simulink model "FMLibrary_v2_progress"  (R2016b)
settings: Solver=VariableStepAuto  StartTime=0.0  StopTime=10.0  RelTol=1e-3
undefined symbols (not defined in the file or in its folder): Lb, Lf, Lu, RobotStruct, sampleTime
libraries: simulink x24, FM_Library x10, VariousBlocksLibrary x10, FMLibrary_v2 x2, simulink_extras x2
(part 2 of 3)

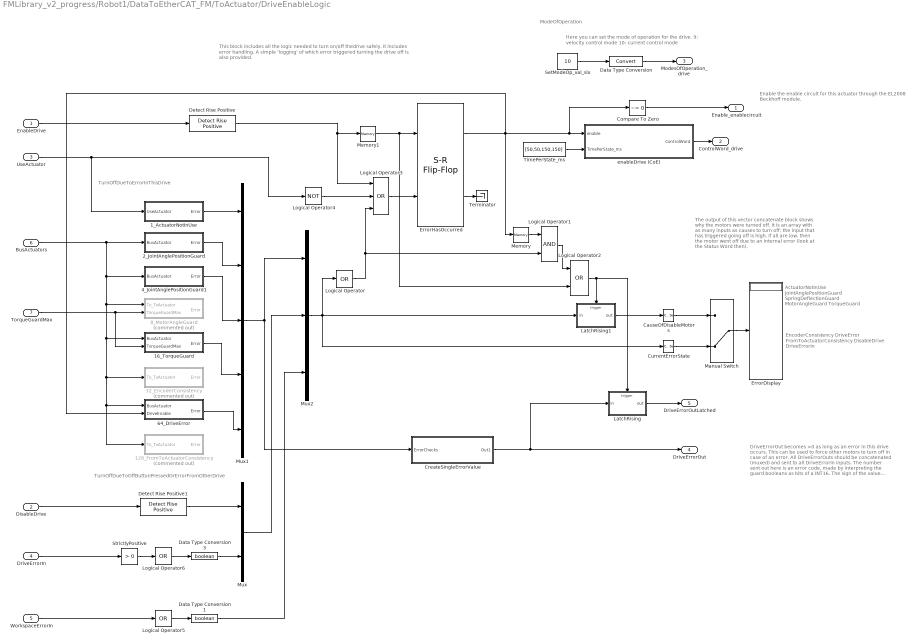
== system FMLibrary_v2_progress/Robot1/DataToEtherCAT_FM/ToActuator/DriveEnableLogic ==
  note: Here you can set the mode of operation for the drive.
      | 9: velocity control mode
      | 10: current control mode
  note: The output of this vector concatenate block shows why the motors were turned off. It is an array with as many inputs as causes to turn off; the input that has triggered going off is high. If all are low, then the motor went off due to an internal error (look at the Status Word then).
  note: This block includes all the logic needed to turn on/off thedrive safely. It includes error handling. A simple 'logging' of which error triggered turning the drive off is also provided.
  note: TurnOffDueToErrorInThisDrive
  note: TurnOffDueToOffButtonPressedOrErrorFromOtherDrive
  note: DriveErrorOut becomes >0 as long as an error in this drive occurs. This can be used to force other motors to turn off in case of an error.
      | All DriveErrorOuts should be concatenated (muxed)  and sent to all DriveErrorIn inputs. The number sent out here is an error code, made by interpreting the guard booleans as bits of a INT16.
      | The sign of the value indicates:
      | >=0: UseActuator=true
      | <0: UseActuator = False
  note: EncoderConsistency
      | DriveError
      | FromToActuatorConsistency
      | DisableDrive
      | DriveErrorIn
  note: ActuatorNotInUse
      | JointAnglePositionGuard
      | SpringDeflectionGuard
      | MotorAngleGuard
      | TorqueGuard
  note: ModeOfOperation
  note: Enable the enable circuit for this actuator through the EL2008
      | Beckhoff module.
  EnableDrive : Inport
  DisableDrive : Inport  Port=2
  UseActuator : Inport  Port=3
  DriveErrorIn : Inport  Port=4
  WorkspaceErrorIn : Inport  Port=5
  BusActuators : Inport  Port=6
  TorqueGuardMax : Inport  Port=7
  128_FromToActuatorConsistency : Subsystem  Commented=on
  16_TorqueGuard : Subsystem
  1_ActuatorNotInUse : Subsystem
  2_JointAnglePositionGuard : Subsystem
  32_EncoderConsistency : Subsystem  Commented=on
  4_JointAnglePositionGuard1 : Subsystem
  64_DriveError : Subsystem
  8_MotorAngleGuard : Subsystem  Commented=on
  CauseOfDisableMotors : Concatenate  NumInputs=1
  Compare To Zero : simulink/Logic and Bit Operations/Compare To Zero  relop=~=  OutDataTypeStr=boolean
  CreateSingleErrorValue : Subsystem
  CurrentErrorState : Concatenate  NumInputs=1
  Data Type Conversion : DataTypeConversion
  Data Type Conversion1 : DataTypeConversion  OutDataTypeStr=boolean
  Data Type Conversion3 : DataTypeConversion  OutDataTypeStr=boolean
  Detect Rise Positive : simulink/Logic and Bit Operations/Detect Rise Positive  vinit=0  InputProcessing=Inherited  OutDataTypeStr=boolean
  Detect Rise Positive1 : simulink/Logic and Bit Operations/Detect Rise Positive  vinit=0  InputProcessing=Inherited  OutDataTypeStr=boolean
  ErrorDisplay : Display
  ErrorHasOccurred : simulink_extras/Flip Flops/S-R Flip-Flop  initial_condition=0
  LatchRising : Subsystem  TreatAsAtomicUnit=on
  LatchRising1 : Subsystem  TreatAsAtomicUnit=on
  Logical Operator : Logic  Operator=OR  Inputs=1  AllPortsSameDT=off  OutDataTypeStr=boolean
  Logical Operator1 : Logic  AllPortsSameDT=off  OutDataTypeStr=boolean
  Logical Operator2 : Logic  Operator=OR  AllPortsSameDT=off  OutDataTypeStr=boolean
  Logical Operator3 : Logic  Operator=OR  Inputs=3  AllPortsSameDT=off  OutDataTypeStr=boolean
  Logical Operator4 : Logic  Operator=NOT  Inputs=1  AllPortsSameDT=off  OutDataTypeStr=boolean
  Logical Operator5 : Logic  Operator=OR  Inputs=1  AllPortsSameDT=off  OutDataTypeStr=boolean
  Logical Operator6 : Logic  Operator=OR  Inputs=1  AllPortsSameDT=off  OutDataTypeStr=boolean
  Manual Switch : ManualSwitch  CurrentSetting=0
  Memory : Memory
  Memory1 : Memory
  Mux : Mux  Inputs=2
  Mux1 : Mux  Inputs=5
  Mux2 : Mux  Inputs=3
  SetModeOp_val_slx : Constant  Value=10
  StrictlyPositive : simulink/Logic and Bit Operations/Compare To Zero  relop=>  OutDataTypeStr=boolean
  Terminator : Terminator
  TimePerState_ms : Constant  Value=[50,50,150,150]
  enableDrive (CoE) : MATLAB Function  TreatAsAtomicUnit=on
  Enable_enablecircuit : Outport
  ControlWord_drive : Outport  Port=2
  ModesOfOperation_drive : Outport  Port=3
  DriveErrorOut : Outport  Port=4
  DriveErrorOutLatched : Outport  Port=5
  wires:
  Data Type Conversion1/1 -> Mux2/3
  Mux1/1 -> Mux2/1, CreateSingleErrorValue/1(ErrorChecks)
  WorkspaceErrorIn/1 -> Logical Operator5/1
  Logical Operator5/1 -> Data Type Conversion1/1
  Data Type Conversion3/1 -> Mux/2
  Compare To Zero/1 -> Enable_enablecircuit/1
  16_TorqueGuard/1(Error) -> Mux1/4
  64_DriveError/1(Error) -> Mux1/5
  1_ActuatorNotInUse/1(Error) -> Mux1/1
  Logical Operator4/1 -> Logical Operator3/2
  BusActuators/1 -> 4_JointAnglePositionGuard1/1(BusActuator), 32_EncoderConsistency/1(To_ToActuator), 64_DriveError/1(BusActuator), 128_FromToActuatorConsistency/1(To_ToActuator), 16_TorqueGuard/1(BusActuator), 8_MotorAngleGuard/1(To_ToActuator), 2_JointAnglePositionGuard/1(BusActuator)
  Mux/1 -> Mux2/2
  Logical Operator6/1 -> Data Type Conversion3/1
  DriveErrorIn/1 -> StrictlyPositive/1
  UseActuator/1 -> Logical Operator4/1, 1_ActuatorNotInUse/1(UseActuator)
  TimePerState_ms/1 -> enableDrive (CoE)/2(TimePerState_ms)
  Detect Rise Positive/1 -> Memory1/1, Logical Operator3/1
  Logical Operator3/1 -> ErrorHasOccurred/2
  Manual Switch/1 -> ErrorDisplay/1
  Logical Operator1/1 -> Logical Operator2/1
  CurrentErrorState/1 -> Manual Switch/2
  Logical Operator2/1 -> LatchRising/Trigger, LatchRising1/Trigger
  Memory/1 -> Logical Operator1/1
  Memory1/1 -> ErrorHasOccurred/1, Logical Operator2/2
  CauseOfDisableMotors/1 -> Manual Switch/1
  Data Type Conversion/1 -> ModesOfOperation_drive/1
  ErrorHasOccurred/2 -> Terminator/1
  DisableDrive/1 -> Detect Rise Positive1/1
  Detect Rise Positive1/1 -> Mux/1
  Mux2/1 -> LatchRising1/1(in), CurrentErrorState/1, Logical Operator/1
  ErrorHasOccurred/1 -> enableDrive (CoE)/1(enable), Compare To Zero/1, 64_DriveError/2(DriveEnable), Memory/1
  enableDrive (CoE)/1(ControlWord) -> ControlWord_drive/1
  EnableDrive/1 -> Detect Rise Positive/1
  SetModeOp_val_slx/1 -> Data Type Conversion/1
  Logical Operator/1 -> Logical Operator1/2, Logical Operator3/3
  LatchRising1/1(out) -> CauseOfDisableMotors/1
  TorqueGuardMax/1 -> 8_MotorAngleGuard/2(TorqueGuardMax), 16_TorqueGuard/2(TorqueGuardMax)
  StrictlyPositive/1 -> Logical Operator6/1
  CreateSingleErrorValue/1(Out1) -> LatchRising/1(in), DriveErrorOut/1
  LatchRising/1(out) -> DriveErrorOutLatched/1
  4_JointAnglePositionGuard1/1(Error) -> Mux1/3
  2_JointAnglePositionGuard/1(Error) -> Mux1/2

== system FMLibrary_v2_progress/Robot1/DataToEtherCAT_FM/ToActuator1/AppendToBus ==
  Bus_in : Inport
  DriveError : Inport  Port=2
  DesiredTorque : Inport  Port=3
  DesiredTorqueLimited : Inport  Port=4
  Bus Creator : BusCreator  Inputs=12
  Bus Selector2 : BusSelector  OutputSignals=OperationEnabled,StatusWord,JointPosition_rad,JointVelocity_rads,MotorEncoder_counts,MotorPosition_IncEnc_rad,JointPosition_IncEnc_rad,JointAbsoluteEncoder_counts,JointTorque_Act_Nm
  Data Type Conversion : DataTypeConversion  OutDataTypeStr=double
  Bus_out : Outport
  wires:
  Bus Selector2/9 -> Bus Creator/9  "<JointTorque_Act_Nm>"
  Bus Creator/1 -> Bus_out/1
  Bus_in/1 -> Bus Selector2/1
  DriveError/1 -> Data Type Conversion/1
  Data Type Conversion/1 -> Bus Creator/12  "DriveError"
  DesiredTorque/1 -> Bus Creator/10  "DesiredTorque_Nm"
  DesiredTorqueLimited/1 -> Bus Creator/11  "DesiredTorqueLimited_Nm"
  Bus Selector2/1 -> Bus Creator/1  "<OperationEnabled>"
  Bus Selector2/2 -> Bus Creator/2  "<StatusWord>"
  Bus Selector2/3 -> Bus Creator/3  "<JointPosition_rad>"
  Bus Selector2/4 -> Bus Creator/4  "<JointVelocity_rads>"
  Bus Selector2/5 -> Bus Creator/5  "<MotorEncoder_counts>"
  Bus Selector2/7 -> Bus Creator/7  "<JointPosition_IncEnc_rad>"
  Bus Selector2/8 -> Bus Creator/8  "<JointAbsoluteEncoder_counts>"
  Bus Selector2/6 -> Bus Creator/6  "<MotorPosition_IncEnc_rad>"

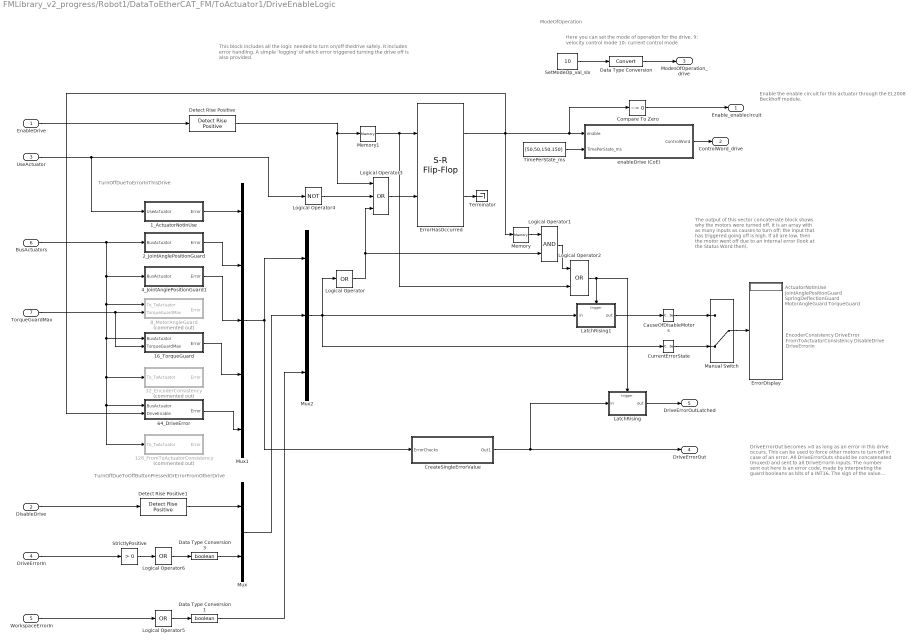
== system FMLibrary_v2_progress/Robot1/DataToEtherCAT_FM/ToActuator1/DriveEnableLogic ==
  note: Here you can set the mode of operation for the drive.
      | 9: velocity control mode
      | 10: current control mode
  note: The output of this vector concatenate block shows why the motors were turned off. It is an array with as many inputs as causes to turn off; the input that has triggered going off is high. If all are low, then the motor went off due to an internal error (look at the Status Word then).
  note: This block includes all the logic needed to turn on/off thedrive safely. It includes error handling. A simple 'logging' of which error triggered turning the drive off is also provided.
  note: TurnOffDueToErrorInThisDrive
  note: TurnOffDueToOffButtonPressedOrErrorFromOtherDrive
  note: DriveErrorOut becomes >0 as long as an error in this drive occurs. This can be used to force other motors to turn off in case of an error.
      | All DriveErrorOuts should be concatenated (muxed)  and sent to all DriveErrorIn inputs. The number sent out here is an error code, made by interpreting the guard booleans as bits of a INT16.
      | The sign of the value indicates:
      | >=0: UseActuator=true
      | <0: UseActuator = False
  note: EncoderConsistency
      | DriveError
      | FromToActuatorConsistency
      | DisableDrive
      | DriveErrorIn
  note: ActuatorNotInUse
      | JointAnglePositionGuard
      | SpringDeflectionGuard
      | MotorAngleGuard
      | TorqueGuard
  note: ModeOfOperation
  note: Enable the enable circuit for this actuator through the EL2008
      | Beckhoff module.
  EnableDrive : Inport
  DisableDrive : Inport  Port=2
  UseActuator : Inport  Port=3
  DriveErrorIn : Inport  Port=4
  WorkspaceErrorIn : Inport  Port=5
  BusActuators : Inport  Port=6
  TorqueGuardMax : Inport  Port=7
  128_FromToActuatorConsistency : Subsystem  Commented=on
  16_TorqueGuard : Subsystem
  1_ActuatorNotInUse : Subsystem
  2_JointAnglePositionGuard : Subsystem
  32_EncoderConsistency : Subsystem  Commented=on
  4_JointAnglePositionGuard1 : Subsystem
  64_DriveError : Subsystem
  8_MotorAngleGuard : Subsystem  Commented=on
  CauseOfDisableMotors : Concatenate  NumInputs=1
  Compare To Zero : simulink/Logic and Bit Operations/Compare To Zero  relop=~=  OutDataTypeStr=boolean
  CreateSingleErrorValue : Subsystem
  CurrentErrorState : Concatenate  NumInputs=1
  Data Type Conversion : DataTypeConversion
  Data Type Conversion1 : DataTypeConversion  OutDataTypeStr=boolean
  Data Type Conversion3 : DataTypeConversion  OutDataTypeStr=boolean
  Detect Rise Positive : simulink/Logic and Bit Operations/Detect Rise Positive  vinit=0  InputProcessing=Inherited  OutDataTypeStr=boolean
  Detect Rise Positive1 : simulink/Logic and Bit Operations/Detect Rise Positive  vinit=0  InputProcessing=Inherited  OutDataTypeStr=boolean
  ErrorDisplay : Display
  ErrorHasOccurred : simulink_extras/Flip Flops/S-R Flip-Flop  initial_condition=0
  LatchRising : Subsystem  TreatAsAtomicUnit=on
  LatchRising1 : Subsystem  TreatAsAtomicUnit=on
  Logical Operator : Logic  Operator=OR  Inputs=1  AllPortsSameDT=off  OutDataTypeStr=boolean
  Logical Operator1 : Logic  AllPortsSameDT=off  OutDataTypeStr=boolean
  Logical Operator2 : Logic  Operator=OR  AllPortsSameDT=off  OutDataTypeStr=boolean
  Logical Operator3 : Logic  Operator=OR  Inputs=3  AllPortsSameDT=off  OutDataTypeStr=boolean
  Logical Operator4 : Logic  Operator=NOT  Inputs=1  AllPortsSameDT=off  OutDataTypeStr=boolean
  Logical Operator5 : Logic  Operator=OR  Inputs=1  AllPortsSameDT=off  OutDataTypeStr=boolean
  Logical Operator6 : Logic  Operator=OR  Inputs=1  AllPortsSameDT=off  OutDataTypeStr=boolean
  Manual Switch : ManualSwitch  CurrentSetting=0
  Memory : Memory
  Memory1 : Memory
  Mux : Mux  Inputs=2
  Mux1 : Mux  Inputs=5
  Mux2 : Mux  Inputs=3
  SetModeOp_val_slx : Constant  Value=10
  StrictlyPositive : simulink/Logic and Bit Operations/Compare To Zero  relop=>  OutDataTypeStr=boolean
  Terminator : Terminator
  TimePerState_ms : Constant  Value=[50,50,150,150]
  enableDrive (CoE) : MATLAB Function  TreatAsAtomicUnit=on
  Enable_enablecircuit : Outport
  ControlWord_drive : Outport  Port=2
  ModesOfOperation_drive : Outport  Port=3
  DriveErrorOut : Outport  Port=4
  DriveErrorOutLatched : Outport  Port=5
  wires:
  Data Type Conversion1/1 -> Mux2/3
  Mux1/1 -> Mux2/1, CreateSingleErrorValue/1(ErrorChecks)
  WorkspaceErrorIn/1 -> Logical Operator5/1
  Logical Operator5/1 -> Data Type Conversion1/1
  Data Type Conversion3/1 -> Mux/2
  Compare To Zero/1 -> Enable_enablecircuit/1
  16_TorqueGuard/1(Error) -> Mux1/4
  64_DriveError/1(Error) -> Mux1/5
  1_ActuatorNotInUse/1(Error) -> Mux1/1
  Logical Operator4/1 -> Logical Operator3/2
  BusActuators/1 -> 4_JointAnglePositionGuard1/1(BusActuator), 32_EncoderConsistency/1(To_ToActuator), 64_DriveError/1(BusActuator), 128_FromToActuatorConsistency/1(To_ToActuator), 16_TorqueGuard/1(BusActuator), 8_MotorAngleGuard/1(To_ToActuator), 2_JointAnglePositionGuard/1(BusActuator)
  Mux/1 -> Mux2/2
  Logical Operator6/1 -> Data Type Conversion3/1
  DriveErrorIn/1 -> StrictlyPositive/1
  UseActuator/1 -> Logical Operator4/1, 1_ActuatorNotInUse/1(UseActuator)
  TimePerState_ms/1 -> enableDrive (CoE)/2(TimePerState_ms)
  Detect Rise Positive/1 -> Memory1/1, Logical Operator3/1
  Logical Operator3/1 -> ErrorHasOccurred/2
  Manual Switch/1 -> ErrorDisplay/1
  Logical Operator1/1 -> Logical Operator2/1
  CurrentErrorState/1 -> Manual Switch/2
  Logical Operator2/1 -> LatchRising/Trigger, LatchRising1/Trigger
  Memory/1 -> Logical Operator1/1
  Memory1/1 -> ErrorHasOccurred/1, Logical Operator2/2
  CauseOfDisableMotors/1 -> Manual Switch/1
  Data Type Conversion/1 -> ModesOfOperation_drive/1
  ErrorHasOccurred/2 -> Terminator/1
  DisableDrive/1 -> Detect Rise Positive1/1
  Detect Rise Positive1/1 -> Mux/1
  Mux2/1 -> LatchRising1/1(in), CurrentErrorState/1, Logical Operator/1
  ErrorHasOccurred/1 -> enableDrive (CoE)/1(enable), Compare To Zero/1, 64_DriveError/2(DriveEnable), Memory/1
  enableDrive (CoE)/1(ControlWord) -> ControlWord_drive/1
  EnableDrive/1 -> Detect Rise Positive/1
  SetModeOp_val_slx/1 -> Data Type Conversion/1
  Logical Operator/1 -> Logical Operator1/2, Logical Operator3/3
  LatchRising1/1(out) -> CauseOfDisableMotors/1
  TorqueGuardMax/1 -> 8_MotorAngleGuard/2(TorqueGuardMax), 16_TorqueGuard/2(TorqueGuardMax)
  StrictlyPositive/1 -> Logical Operator6/1
  CreateSingleErrorValue/1(Out1) -> LatchRising/1(in), DriveErrorOut/1
  LatchRising/1(out) -> DriveErrorOutLatched/1
  4_JointAnglePositionGuard1/1(Error) -> Mux1/3
  2_JointAnglePositionGuard/1(Error) -> Mux1/2

== system FMLibrary_v2_progress/Robot1/DataToEtherCAT_FM/WorkspacePositionGuard/CreateSingleErrorValue ==
  ErrorChecks : Inport
  Data Type Conversion1 : DataTypeConversion  OutDataTypeStr=double
  Data Type Conversion2 : DataTypeConversion  OutDataTypeStr=int32
  MATLAB Function : MATLAB Function  TreatAsAtomicUnit=on
  error : Outport
  wires:
  Data Type Conversion2/1 -> error/1
  ErrorChecks/1 -> Data Type Conversion1/1
  Data Type Conversion1/1 -> MATLAB Function/1(errors)
  MATLAB Function/1(out) -> Data Type Conversion2/1

== system FMLibrary_v2_progress/Robot1/DataToEtherCAT_FM/ToActuator/DriveEnableLogic/128_FromToActuatorConsistency ==
  note: This block checks whether the FromActuator and ToActuator blocks use the same ActuatorStruct. If not, you've done something wrong. It does this by checking if the JointEncoderOffsets are identical.
  To_ToActuator : Inport
  Bus Selector : BusSelector  OutputSignals=JointEncoderOffset
  Constant : Constant  Value=ActuatorStruct.JointEncoderOffset
  Relational Operator : RelationalOperator  Operator=~=  OutDataTypeStr=boolean  RndMeth=Nearest
  Error : Outport
  wires:
  Constant/1 -> Relational Operator/2
  Bus Selector/1 -> Relational Operator/1  "<JointEncoderOffset>"
  Relational Operator/1 -> Error/1
  To_ToActuator/1 -> Bus Selector/1

== system FMLibrary_v2_progress/Robot1/DataToEtherCAT_FM/ToActuator/DriveEnableLogic/16_TorqueGuard ==
  BusActuator : Inport
  TorqueGuardMax : Inport  Port=2
  Abs : Abs
  Bus Selector : BusSelector  OutputSignals=JointTorque_Act_Nm
  Relational Operator : RelationalOperator  Operator=>  OutDataTypeStr=boolean  RndMeth=Nearest
  Error : Outport  PortDimensions=1
  wires:
  Relational Operator/1 -> Error/1
  Abs/1 -> Relational Operator/1
  BusActuator/1 -> Bus Selector/1
  Bus Selector/1 -> Abs/1  "<JointTorque_Act_Nm>"
  TorqueGuardMax/1 -> Relational Operator/2

== system FMLibrary_v2_progress/Robot1/DataToEtherCAT_FM/ToActuator/DriveEnableLogic/1_ActuatorNotInUse ==
  note: When UseActuator = 0, this block outputs 1. Later in the chain, the ErrorValue is then negated, resulting in -1 if there are no other errors. Note, thus, that this output does not really indicate an error; more a status.
  UseActuator : Inport
  Logical Operator1 : Logic  Operator=NOT  AllPortsSameDT=off  OutDataTypeStr=boolean
  Error : Outport  PortDimensions=1
  wires:
  UseActuator/1 -> Logical Operator1/1
  Logical Operator1/1 -> Error/1

== system FMLibrary_v2_progress/Robot1/DataToEtherCAT_FM/ToActuator/DriveEnableLogic/2_JointAnglePositionGuard ==
  note: This block makes sure that the motors are turned off (and cannot go on) when the joint is outside its normal range.
  BusActuator : Inport
  Bus Selector : BusSelector  OutputSignals=JointPosition_rad
  Logical Operator : Logic  Operator=OR  AllPortsSameDT=off  OutDataTypeStr=boolean
  Maximum : Constant  Value=ActuatorStruct.JointPositionGuardMax
  Minimum : Constant  Value=ActuatorStruct.JointPositionGuardMin
  Relational Operator : RelationalOperator  Operator=<=  OutDataTypeStr=boolean  RndMeth=Nearest
  Relational Operator1 : RelationalOperator  OutDataTypeStr=boolean  RndMeth=Nearest
  Error : Outport
  wires:
  Bus Selector/1 -> Relational Operator/1, Relational Operator1/1  "<JointPosition_rad>"
  Maximum/1 -> Relational Operator1/2
  Minimum/1 -> Relational Operator/2
  Logical Operator/1 -> Error/1
  Relational Operator1/1 -> Logical Operator/2
  Relational Operator/1 -> Logical Operator/1
  BusActuator/1 -> Bus Selector/1

== system FMLibrary_v2_progress/Robot1/DataToEtherCAT_FM/ToActuator/DriveEnableLogic/32_EncoderConsistency ==
  note: This block checks whether the three encoders are consistent. Ideally, the sum (with jointAngle negated) should be exactly zero at all times (also when forces are exerted). We allow some room around it however.
  To_ToActuator : Inport
  Abs : Abs
  Add : Sum  Inputs=+-
  Bus Selector : BusSelector  OutputSignals=JointPosition_IncEnc_rad,JointPosition_AbsEnc_rad
  Compare To Constant : simulink/Logic and Bit Operations/Compare To Constant  relop=<=  const=3.0  OutDataTypeStr=boolean
  EncoderInConsistency_rad : Concatenate  NumInputs=1
  Error : Outport
  wires:
  EncoderInConsistency_rad/1 -> Abs/1
  Add/1 -> EncoderInConsistency_rad/1
  Bus Selector/2 -> Add/2  "<JointPosition_AbsEnc_rad>"
  Abs/1 -> Compare To Constant/1
  Compare To Constant/1 -> Error/1
  To_ToActuator/1 -> Bus Selector/1
  Bus Selector/1 -> Add/1  "<JointPosition_IncEnc_rad>"

== system FMLibrary_v2_progress/Robot1/DataToEtherCAT_FM/ToActuator/DriveEnableLogic/4_JointAnglePositionGuard1 ==
  note: This block makes sure that the motors are turned off when the transmission slips.
  BusActuator : Inport
  Bus Selector : BusSelector  OutputSignals=JointPosition_rad,JointPosition_IncEnc_rad
  Minimum : Constant  Value=ActuatorStruct.TransmissionSlipAngleGuardMax
  Relational Operator1 : RelationalOperator  OutDataTypeStr=boolean  RndMeth=Nearest
  Subtract : Sum  Inputs=+-
  Error : Outport
  wires:
  Bus Selector/1 -> Subtract/1  "<JointPosition_rad>"
  Relational Operator1/1 -> Error/1
  BusActuator/1 -> Bus Selector/1
  Minimum/1 -> Relational Operator1/2
  Bus Selector/2 -> Subtract/2  "<JointPosition_IncEnc_rad>"
  Subtract/1 -> Relational Operator1/1

== system FMLibrary_v2_progress/Robot1/DataToEtherCAT_FM/ToActuator/DriveEnableLogic/64_DriveError ==
  note: This block checks whether the drive went off by itself. Reasons why this could happen are: undervoltage of the motor power supply, short-circuit detection triggered, I2t error etc.
      | The first few seconds that the drive should be on (i.e., DriveEnable = True), the drive is in the process of turning on, and will not be really on. In order to avoid direct turn-off due to this, we disable this error the first few seconds.
  note: This memory block is to avoid an
      | algebraic loop
  note: This memory block is to avoid that this error 'turns on' when another error is triggered.
  BusActuator : Inport
  DriveEnable : Inport  Port=2
  Bus Selector : BusSelector  OutputSignals=OperationEnabled
  CountHowLongEnableWasTrue : MATLAB Function  TreatAsAtomicUnit=on
  InhibitTime_s : Constant  Value=2.0
  Logical Operator : Logic  AllPortsSameDT=off  OutDataTypeStr=boolean
  Logical Operator2 : Logic  Operator=NOT  AllPortsSameDT=off  OutDataTypeStr=boolean
  Memory : Memory
  Memory1 : Memory
  Relational Operator : RelationalOperator  OutDataTypeStr=boolean  RndMeth=Nearest
  ToSeconds : Gain  Gain=sampleTime
  Error : Outport  PortDimensions=1
  wires:
  Logical Operator2/1 -> Logical Operator/2
  Memory1/1 -> Bus Selector/1
  Memory/1 -> CountHowLongEnableWasTrue/1(u)
  InhibitTime_s/1 -> Relational Operator/2
  Relational Operator/1 -> Logical Operator/1
  ToSeconds/1 -> Relational Operator/1
  CountHowLongEnableWasTrue/1(y) -> ToSeconds/1
  DriveEnable/1 -> Memory/1
  Bus Selector/1 -> Logical Operator2/1  "<OperationEnabled>"
  BusActuator/1 -> Memory1/1
  Logical Operator/1 -> Error/1

== system FMLibrary_v2_progress/Robot1/DataToEtherCAT_FM/ToActuator/DriveEnableLogic/8_MotorAngleGuard ==
  note: This block checks whether the motor encoder gives sensible data, i.e., if the motor angle is within the expected range. The expected range is the full stroke of the output shaft plus the maximum spring deflection, transformed to motor angle space.
  To_ToActuator : Inport
  TorqueGuardMax : Inport  Port=2
  Add : Sum  Inputs=+-
  Add1 : Sum
  Bus Selector : BusSelector  OutputSignals=MotorPosition_IncEnc_rad
  Divide : Product  Inputs=*/
  Logical Operator : Logic  Operator=OR  AllPortsSameDT=off  OutDataTypeStr=boolean
  Maximum : Constant  Value=ActuatorStruct.JointAnglePositionGuardMax_rad
  Minimum : Constant  Value=ActuatorStruct.JointAnglePositionGuardMin_rad
  Relational Operator1 : RelationalOperator  Operator=<=  OutDataTypeStr=boolean  RndMeth=Nearest
  Relational Operator2 : RelationalOperator  OutDataTypeStr=boolean  RndMeth=Nearest
  SpringStiffness : Constant  Value=ActuatorStruct.SpringStiffness_Nm_rad
  TransformToMotorSpace : Gain  Gain=ActuatorStruct.gearboxRatio
  TransformToMotorSpace1 : Gain  Gain=ActuatorStruct.gearboxRatio
  Error : Outport
  wires:
  Minimum/1 -> Add/1
  Divide/1 -> Add1/2, Add/2  "MaximumSpringDeflection_rad"
  Maximum/1 -> Add1/1
  SpringStiffness/1 -> Divide/2
  TorqueGuardMax/1 -> Divide/1
  TransformToMotorSpace/1 -> Relational Operator2/2
  Add/1 -> TransformToMotorSpace1/1
  Add1/1 -> TransformToMotorSpace/1
  TransformToMotorSpace1/1 -> Relational Operator1/2
  Logical Operator/1 -> Error/1
  Relational Operator2/1 -> Logical Operator/2
  Relational Operator1/1 -> Logical Operator/1
  Bus Selector/1 -> Relational Operator1/1, Relational Operator2/1  "<MotorPosition_IncEnc_rad>"
  To_ToActuator/1 -> Bus Selector/1

== system FMLibrary_v2_progress/Robot1/DataToEtherCAT_FM/ToActuator/DriveEnableLogic/CreateSingleErrorValue ==
  ErrorChecks : Inport
  Data Type Conversion1 : DataTypeConversion  OutDataTypeStr=double
  Data Type Conversion2 : DataTypeConversion  OutDataTypeStr=int32
  MATLAB Function : MATLAB Function  TreatAsAtomicUnit=on
  Select_NotUseActuator : Selector  InputPortWidth=3  IndexOptions=Index vector (dialog)  Indices=1  OutputSizes=1
  Switch : Switch  Criteria=u2 ~= 0
  Unary Minus : UnaryMinus
  Out1 : Outport
  wires:
  Unary Minus/1 -> Switch/1
  Switch/1 -> Out1/1
  ErrorChecks/1 -> Data Type Conversion1/1
  Select_NotUseActuator/1 -> Switch/2
  Data Type Conversion1/1 -> Select_NotUseActuator/1, MATLAB Function/1(errors)
  MATLAB Function/1(out) -> Data Type Conversion2/1
  Data Type Conversion2/1 -> Unary Minus/1, Switch/3

== system FMLibrary_v2_progress/Robot1/DataToEtherCAT_FM/ToActuator/DriveEnableLogic/LatchRising ==
  in : Inport
  Trigger : TriggerPort  VariantControl=Variant  PortDimensions=1
  out : Outport
  wires:
  in/1 -> out/1

== system FMLibrary_v2_progress/Robot1/DataToEtherCAT_FM/ToActuator/DriveEnableLogic/LatchRising1 ==
  in : Inport
  Trigger : TriggerPort  VariantControl=Variant  PortDimensions=1
  out : Outport
  wires:
  in/1 -> out/1

== system FMLibrary_v2_progress/Robot1/DataToEtherCAT_FM/ToActuator1/DriveEnableLogic/128_FromToActuatorConsistency ==
  note: This block checks whether the FromActuator and ToActuator blocks use the same ActuatorStruct. If not, you've done something wrong. It does this by checking if the JointEncoderOffsets are identical.
  To_ToActuator : Inport
  Bus Selector : BusSelector  OutputSignals=JointEncoderOffset
  Constant : Constant  Value=ActuatorStruct.JointEncoderOffset
  Relational Operator : RelationalOperator  Operator=~=  OutDataTypeStr=boolean  RndMeth=Nearest
  Error : Outport
  wires:
  Constant/1 -> Relational Operator/2
  Bus Selector/1 -> Relational Operator/1  "<JointEncoderOffset>"
  Relational Operator/1 -> Error/1
  To_ToActuator/1 -> Bus Selector/1

== system FMLibrary_v2_progress/Robot1/DataToEtherCAT_FM/ToActuator1/DriveEnableLogic/16_TorqueGuard ==
  BusActuator : Inport
  TorqueGuardMax : Inport  Port=2
  Abs : Abs
  Bus Selector : BusSelector  OutputSignals=JointTorque_Act_Nm
  Relational Operator : RelationalOperator  Operator=>  OutDataTypeStr=boolean  RndMeth=Nearest
  Error : Outport  PortDimensions=1
  wires:
  Relational Operator/1 -> Error/1
  Abs/1 -> Relational Operator/1
  BusActuator/1 -> Bus Selector/1
  Bus Selector/1 -> Abs/1  "<JointTorque_Act_Nm>"
  TorqueGuardMax/1 -> Relational Operator/2

== system FMLibrary_v2_progress/Robot1/DataToEtherCAT_FM/ToActuator1/DriveEnableLogic/1_ActuatorNotInUse ==
  note: When UseActuator = 0, this block outputs 1. Later in the chain, the ErrorValue is then negated, resulting in -1 if there are no other errors. Note, thus, that this output does not really indicate an error; more a status.
  UseActuator : Inport
  Logical Operator1 : Logic  Operator=NOT  AllPortsSameDT=off  OutDataTypeStr=boolean
  Error : Outport  PortDimensions=1
  wires:
  UseActuator/1 -> Logical Operator1/1
  Logical Operator1/1 -> Error/1

== system FMLibrary_v2_progress/Robot1/DataToEtherCAT_FM/ToActuator1/DriveEnableLogic/2_JointAnglePositionGuard ==
  note: This block makes sure that the motors are turned off (and cannot go on) when the joint is outside its normal range.
  BusActuator : Inport
  Bus Selector : BusSelector  OutputSignals=JointPosition_rad
  Logical Operator : Logic  Operator=OR  AllPortsSameDT=off  OutDataTypeStr=boolean
  Maximum : Constant  Value=ActuatorStruct.JointPositionGuardMax
  Minimum : Constant  Value=ActuatorStruct.JointPositionGuardMin
  Relational Operator : RelationalOperator  Operator=<=  OutDataTypeStr=boolean  RndMeth=Nearest
  Relational Operator1 : RelationalOperator  OutDataTypeStr=boolean  RndMeth=Nearest
  Error : Outport
  wires:
  Bus Selector/1 -> Relational Operator/1, Relational Operator1/1  "<JointPosition_rad>"
  Maximum/1 -> Relational Operator1/2
  Minimum/1 -> Relational Operator/2
  Logical Operator/1 -> Error/1
  Relational Operator1/1 -> Logical Operator/2
  Relational Operator/1 -> Logical Operator/1
  BusActuator/1 -> Bus Selector/1

== system FMLibrary_v2_progress/Robot1/DataToEtherCAT_FM/ToActuator1/DriveEnableLogic/32_EncoderConsistency ==
  note: This block checks whether the three encoders are consistent. Ideally, the sum (with jointAngle negated) should be exactly zero at all times (also when forces are exerted). We allow some room around it however.
  To_ToActuator : Inport
  Abs : Abs
  Add : Sum  Inputs=+-
  Bus Selector : BusSelector  OutputSignals=JointPosition_IncEnc_rad,JointPosition_AbsEnc_rad
  Compare To Constant : simulink/Logic and Bit Operations/Compare To Constant  relop=<=  const=3.0  OutDataTypeStr=boolean
  EncoderInConsistency_rad : Concatenate  NumInputs=1
  Error : Outport
  wires:
  EncoderInConsistency_rad/1 -> Abs/1
  Add/1 -> EncoderInConsistency_rad/1
  Bus Selector/2 -> Add/2  "<JointPosition_AbsEnc_rad>"
  Abs/1 -> Compare To Constant/1
  Compare To Constant/1 -> Error/1
  To_ToActuator/1 -> Bus Selector/1
  Bus Selector/1 -> Add/1  "<JointPosition_IncEnc_rad>"

== system FMLibrary_v2_progress/Robot1/DataToEtherCAT_FM/ToActuator1/DriveEnableLogic/4_JointAnglePositionGuard1 ==
  note: This block makes sure that the motors are turned off when the transmission slips.
  BusActuator : Inport
  Bus Selector : BusSelector  OutputSignals=JointPosition_rad,JointPosition_IncEnc_rad
  Minimum : Constant  Value=ActuatorStruct.TransmissionSlipAngleGuardMax
  Relational Operator1 : RelationalOperator  OutDataTypeStr=boolean  RndMeth=Nearest
  Subtract : Sum  Inputs=+-
  Error : Outport
  wires:
  Bus Selector/1 -> Subtract/1  "<JointPosition_rad>"
  Relational Operator1/1 -> Error/1
  BusActuator/1 -> Bus Selector/1
  Minimum/1 -> Relational Operator1/2
  Bus Selector/2 -> Subtract/2  "<JointPosition_IncEnc_rad>"
  Subtract/1 -> Relational Operator1/1

== system FMLibrary_v2_progress/Robot1/DataToEtherCAT_FM/ToActuator1/DriveEnableLogic/64_DriveError ==
  note: This block checks whether the drive went off by itself. Reasons why this could happen are: undervoltage of the motor power supply, short-circuit detection triggered, I2t error etc.
      | The first few seconds that the drive should be on (i.e., DriveEnable = True), the drive is in the process of turning on, and will not be really on. In order to avoid direct turn-off due to this, we disable this error the first few seconds.
  note: This memory block is to avoid an
      | algebraic loop
  note: This memory block is to avoid that this error 'turns on' when another error is triggered.
  BusActuator : Inport
  DriveEnable : Inport  Port=2
  Bus Selector : BusSelector  OutputSignals=OperationEnabled
  CountHowLongEnableWasTrue : MATLAB Function  TreatAsAtomicUnit=on
  InhibitTime_s : Constant  Value=2.0
  Logical Operator : Logic  AllPortsSameDT=off  OutDataTypeStr=boolean
  Logical Operator2 : Logic  Operator=NOT  AllPortsSameDT=off  OutDataTypeStr=boolean
  Memory : Memory
  Memory1 : Memory
  Relational Operator : RelationalOperator  OutDataTypeStr=boolean  RndMeth=Nearest
  ToSeconds : Gain  Gain=sampleTime
  Error : Outport  PortDimensions=1
  wires:
  Logical Operator2/1 -> Logical Operator/2
  Memory1/1 -> Bus Selector/1
  Memory/1 -> CountHowLongEnableWasTrue/1(u)
  InhibitTime_s/1 -> Relational Operator/2
  Relational Operator/1 -> Logical Operator/1
  ToSeconds/1 -> Relational Operator/1
  CountHowLongEnableWasTrue/1(y) -> ToSeconds/1
  DriveEnable/1 -> Memory/1
  Bus Selector/1 -> Logical Operator2/1  "<OperationEnabled>"
  BusActuator/1 -> Memory1/1
  Logical Operator/1 -> Error/1

== system FMLibrary_v2_progress/Robot1/DataToEtherCAT_FM/ToActuator1/DriveEnableLogic/8_MotorAngleGuard ==
  note: This block checks whether the motor encoder gives sensible data, i.e., if the motor angle is within the expected range. The expected range is the full stroke of the output shaft plus the maximum spring deflection, transformed to motor angle space.
  To_ToActuator : Inport
  TorqueGuardMax : Inport  Port=2
  Add : Sum  Inputs=+-
  Add1 : Sum
  Bus Selector : BusSelector  OutputSignals=MotorPosition_IncEnc_rad
  Divide : Product  Inputs=*/
  Logical Operator : Logic  Operator=OR  AllPortsSameDT=off  OutDataTypeStr=boolean
  Maximum : Constant  Value=ActuatorStruct.JointAnglePositionGuardMax_rad
  Minimum : Constant  Value=ActuatorStruct.JointAnglePositionGuardMin_rad
  Relational Operator1 : RelationalOperator  Operator=<=  OutDataTypeStr=boolean  RndMeth=Nearest
  Relational Operator2 : RelationalOperator  OutDataTypeStr=boolean  RndMeth=Nearest
  SpringStiffness : Constant  Value=ActuatorStruct.SpringStiffness_Nm_rad
  TransformToMotorSpace : Gain  Gain=ActuatorStruct.gearboxRatio
  TransformToMotorSpace1 : Gain  Gain=ActuatorStruct.gearboxRatio
  Error : Outport
  wires:
  Minimum/1 -> Add/1
  Divide/1 -> Add1/2, Add/2  "MaximumSpringDeflection_rad"
  Maximum/1 -> Add1/1
  SpringStiffness/1 -> Divide/2
  TorqueGuardMax/1 -> Divide/1
  TransformToMotorSpace/1 -> Relational Operator2/2
  Add/1 -> TransformToMotorSpace1/1
  Add1/1 -> TransformToMotorSpace/1
  TransformToMotorSpace1/1 -> Relational Operator1/2
  Logical Operator/1 -> Error/1
  Relational Operator2/1 -> Logical Operator/2
  Relational Operator1/1 -> Logical Operator/1
  Bus Selector/1 -> Relational Operator1/1, Relational Operator2/1  "<MotorPosition_IncEnc_rad>"
  To_ToActuator/1 -> Bus Selector/1

== system FMLibrary_v2_progress/Robot1/DataToEtherCAT_FM/ToActuator1/DriveEnableLogic/CreateSingleErrorValue ==
  ErrorChecks : Inport
  Data Type Conversion1 : DataTypeConversion  OutDataTypeStr=double
  Data Type Conversion2 : DataTypeConversion  OutDataTypeStr=int32
  MATLAB Function : MATLAB Function  TreatAsAtomicUnit=on
  Select_NotUseActuator : Selector  InputPortWidth=3  IndexOptions=Index vector (dialog)  Indices=1  OutputSizes=1
  Switch : Switch  Criteria=u2 ~= 0
  Unary Minus : UnaryMinus
  Out1 : Outport
  wires:
  Unary Minus/1 -> Switch/1
  Switch/1 -> Out1/1
  ErrorChecks/1 -> Data Type Conversion1/1
  Select_NotUseActuator/1 -> Switch/2
  Data Type Conversion1/1 -> Select_NotUseActuator/1, MATLAB Function/1(errors)
  MATLAB Function/1(out) -> Data Type Conversion2/1
  Data Type Conversion2/1 -> Unary Minus/1, Switch/3

== system FMLibrary_v2_progress/Robot1/DataToEtherCAT_FM/ToActuator1/DriveEnableLogic/LatchRising ==
  in : Inport
  Trigger : TriggerPort  VariantControl=Variant  PortDimensions=1
  out : Outport
  wires:
  in/1 -> out/1

== system FMLibrary_v2_progress/Robot1/DataToEtherCAT_FM/ToActuator1/DriveEnableLogic/LatchRising1 ==
  in : Inport
  Trigger : TriggerPort  VariantControl=Variant  PortDimensions=1
  out : Outport
  wires:
  in/1 -> out/1

== matlab function FMLibrary_v2_progress/Robot1/DataFromEtherCAT_FM/FromActuator2/CalculateJointVelocity/FOAW ==
  data: x input; xdot output; sampleTime parameter; noise input
function xdot = foaw(x, sampleTime, noise)
%#codegen

SIZE = 100; % number of samples in buffer
NOISE = noise;
Ts = sampleTime;

persistent posbuffer;
persistent buffercntr;

% initialize buffer
if isempty(posbuffer)
    posbuffer = zeros(SIZE,1); % 1D case for now
    buffercntr = 0;
end

% fill buffer: shift data and add new value (loose oldest sample)
posbuffer = [posbuffer(2:end); x];
buffercntr = buffercntr + 1;
if buffercntr > SIZE, buffercntr = SIZE; end;

% if buffercntr = 1, only 1 data point is available, and you can't make a
% velocity prediction based on 1 data point. Set velocity ot 0, and return
% function
xdot = 0;
if buffercntr <= 3
    return;
end

for n = 1:buffercntr-1 % n = window size
        
    % step 2
    currentpos = posbuffer(end);

    % step 3 - calculate LS approximation of slope (hence velocity)
    b = n*sum(posbuffer(end-n:end)) - 2*sum(posbuffer(end-n:end).*(n:-1:0)');
    b = b / (Ts*n*(n+1)*(n+2)/6);

    % step 4 - check whether the line an + bn*Ts passes through all points inside the 
    % window within the uncertainty band of each point 
    jj = 0:n;
    yk_hat = currentpos-(b*jj*Ts);
    yk = posbuffer(end-jj)';
    if any(abs(yk_hat-yk) > NOISE)
        break;
    end

    xdot = b;
end

== matlab function FMLibrary_v2_progress/Robot1/DataFromEtherCAT_FM/FromActuator1/CalculateJointVelocity/FOAW ==
  data: x input; xdot output; sampleTime parameter; noise input
function xdot = foaw(x, sampleTime, noise)
%#codegen

SIZE = 100; % number of samples in buffer
NOISE = noise;
Ts = sampleTime;

persistent posbuffer;
persistent buffercntr;

% initialize buffer
if isempty(posbuffer)
    posbuffer = zeros(SIZE,1); % 1D case for now
    buffercntr = 0;
end

% fill buffer: shift data and add new value (loose oldest sample)
posbuffer = [posbuffer(2:end); x];
buffercntr = buffercntr + 1;
if buffercntr > SIZE, buffercntr = SIZE; end;

% if buffercntr = 1, only 1 data point is available, and you can't make a
% velocity prediction based on 1 data point. Set velocity ot 0, and return
% function
xdot = 0;
if buffercntr <= 3
    return;
end

for n = 1:buffercntr-1 % n = window size
        
    % step 2
    currentpos = posbuffer(end);

    % step 3 - calculate LS approximation of slope (hence velocity)
    b = n*sum(posbuffer(end-n:end)) - 2*sum(posbuffer(end-n:end).*(n:-1:0)');
    b = b / (Ts*n*(n+1)*(n+2)/6);

    % step 4 - check whether the line an + bn*Ts passes through all points inside the 
    % window within the uncertainty band of each point 
    jj = 0:n;
    yk_hat = currentpos-(b*jj*Ts);
    yk = posbuffer(end-jj)';
    if any(abs(yk_hat-yk) > NOISE)
        break;
    end

    xdot = b;
end

== matlab function FMLibrary_v2_progress/Robot1/DataToEtherCAT_FM/FTSensorError/MATLAB Function ==
  data: ForcesTorques input; e output; MaxForcesTorques input
function e = fcn(ForcesTorques, MaxForcesTorques)

% throw error when any of the forces/torques go over a max allowable value
if any(abs(ForcesTorques) > MaxForcesTorques) 
    e = 1;
else
    e = 0;
end

== matlab function FMLibrary_v2_progress/Robot1/DataFromEtherCAT_FM/FromActuator2/CalibrateAbsEncoder ==
  data: encoderPosition input; JointPosition_AbsEnc_rad output; offset input
function JointPosition_AbsEnc_rad = CalibrateAbsoluteEncoder(encoderPosition, offset)
%#codegen

% unwrap encoder angle (in case the encoder goes through 0
encoderPosition = unwrap(encoderPosition);

% remove offset
JointPosition_AbsEnc_rad = encoderPosition - offset;

% since the absolute encoder is mounted upside-down, negate the
% jointposition angle
JointPosition_AbsEnc_rad = -JointPosition_AbsEnc_rad;

== matlab function FMLibrary_v2_progress/Robot1/DataFromEtherCAT_FM/FromActuator2/CalibrateMotorPosition     ==
  data: JointPosition_IncEnc_rad output; MotorPosition_rad input; MotorPositionCalibrated_rad output; transmissionRatio parameter; JointPosition_AbsEnc_rad input; Calibrate input
function [JointPosition_IncEnc_rad,MotorPositionCalibrated_rad]...
    = CalibrateMotorPosition( MotorPosition_rad, transmissionRatio, JointPosition_AbsEnc_rad, Calibrate)
%#codegen

% This block includes calibration such that (ideally) the motor angle is
% zero when the joint angle and spring deflection are zero as well. Before
% the calibration has occurred, the output of this function is -1e9*. This
% is chosen such that the value is always outside the allowed motor angle
% range; this prevents the drive from being allowed to turn on.
% 
% * I wanted to use -inf as starting function, but I'm not sure whether
%   that will be handled correctly in all cases.

persistent isCalibrated;
persistent offset;

if isempty(isCalibrated) % no calibration needed
    isCalibrated = 1;
    offset = 0;
end;


if Calibrate
%     if ~isempty(JointPosition_AbsEnc_rad)
        target_pos_mot_rad = transmissionRatio * JointPosition_AbsEnc_rad; % This is what we should read
%         target_pos_mot_rad = CalibrationAngle; % This is what we should read / fix for now
        offset = target_pos_mot_rad - MotorPosition_rad; % calculate offset
%     else
%         % no absolute encoder data available, offset is zero
%         offset = 0;
%     end
    isCalibrated = 1;
end;

% if already calibrated, calculate calibrated motor angle
if isCalibrated
    MotorPositionCalibrated_rad = MotorPosition_rad + offset;
    JointPosition_IncEnc_rad = MotorPositionCalibrated_rad / transmissionRatio;
else
    MotorPositionCalibrated_rad = MotorPosition_rad;
    JointPosition_IncEnc_rad = MotorPositionCalibrated_rad / transmissionRatio;
end;

== matlab function FMLibrary_v2_progress/Robot1/DataFromEtherCAT_FM/FromActuator2/CheckOperationEnabled ==
  data: u input; y output
function y = fcn(u)
%#codegen

mask  = bin2dec('0000000001101111');
match = bin2dec('0000000000100111');

masked = bitand(u,mask);
if masked==match
    y=1;
else
    y=0;
end;

== matlab function FMLibrary_v2_progress/Robot1/Controller/PD + Nonlinear ID/AFFC/AFFC ==
  data: p output; t input; q input; qdot input; qddot input; e input; tau output; Lf parameter; Lu parameter; Lb parameter; w input
function [p,tau] = fcn(t, q, qdot, qddot, e, Lf, Lu, Lb,w)

persistent p_;

if isempty(p_)
%     p_ = [0.00173;0.00159;0.048;0.07889;-0.00389;0.08784;-0.00474];
    p_ = zeros(7,1);
end


% inverse kinematics & jacobians
% q = func_eq_IK(x(1),x(2),Lf,Lu,Lb);
J = func_eq_Je(q(1),q(2),Lf,Lu,Lb);
% qdot = pinv(J)*xdot;
Jdot = func_eq_Jedot(q(1),q(2),qdot(1),qdot(2),Lf,Lu,Lb);
% qddot = pinv(J)*(xddot-Jdot*qdot);

% create Psi
Psi = [diag([qddot(1) qddot(2)]) J'*J*qddot+J'*Jdot*qdot [sign(qdot(1)) qdot(1); 0 0] [0 0;sign(qdot(2)) qdot(2)] ];

% learning matrix Gamma
eta = 0.95*exp(-t/150) + 0.05;
% eta = 1;
% wI = 1e-3;
% wme = 5e-2;
% wfd = 1e-3;
% wfs = 1e-3;

wI = w(1);
wme = w(2);
wfd = w(3);
wfs = w(4);

Gamma = eta*diag([wI wI wme wfs wfd wfs wfd]);

% update p (parameter vector)

% learning rule
dp = Gamma*Psi'*e;

p_ = p_ + dp;

% Psi = [diag([qddot(1) qddot(2)]) J'*J*qddot+J'*Jdot*qdot [ssign(qdot(1)) qdot(1); 0 0] [0 0;ssign(qdot(2)) qdot(2)] ];


% feedforward torque
tau = Psi*p_;

p = p_;

function y = ssign(u,beta)

if nargin == 1
    beta = 150;
end

y = 2./(1+exp(-beta*u))-1;

== stateflow chart FMLibrary_v2_progress/Robot1/StateMachineLocal/SystemLocalStateMachine ==
  settings: initializeOutput=1
  state Operational
    state Calibration
      en:
      systemState = 2;
      velBelowThreshold = false;
      du:
      velBelowThreshold = checkVelThreshold(0.001 );
      state JointVelLarge
      state JointVelSmall
      state DoCalibration
        en: systemState = 201;
      state CalibrationDone
        en: systemState = 299;
      (default) -> JointVelLarge
      JointVelSmall -> JointVelLarge [order 1] : [!velBelowThreshold]
      JointVelLarge -> JointVelSmall : [velBelowThreshold]
      JointVelSmall -> DoCalibration [order 2] : after(2,sec)
      DoCalibration -> CalibrationDone
    state Homing
      en:
      systemState = reqSystemState;
      isAtHome = false;
      du:
      isAtHome = checkEndpointPosition(homeLocationSize);
      state NotAtHome
      state AtHome
      state HomingDone
        en: systemState = 399;
      (default) -> NotAtHome
      AtHome -> NotAtHome [order 1] : [!isAtHome]
      NotAtHome -> AtHome : [isAtHome]
      AtHome -> HomingDone [order 2] : after(1,sec)
    state Run
      en: systemState = 4;
    (default) -> Calibration
    CalibrationDone -> Homing : [reqSystemState == 301 || reqSystemState == 302]
    Run -> Homing : [reqSystemState==3]
    HomingDone -> Run : [reqSystemState==4]
  state Idle
    en:
    systemState = 0;
  state Init
    en:
    systemState = 1;
    du:
    isInitialized = true;
  state Error
    en: systemState=-1;
  (default) -> Idle
  Init -> Operational [order 1] : [isInitialized]
  Idle -> Init [order 2] : [reqSystemState==1]
  Init -> Idle [order 3] : [reqSystemState==0]
  Error -> Idle : [!error   && reqSystemState==0]
  Init -> Error [order 2] : [error]
  Idle -> Error [order 1] : [error]
  Operational -> Idle [order 2] : [reqSystemState==0]
  Operational -> Error [order 1] : [error]
  data: threshold function_input double; velIsUnderThreshold function_output boolean; threshold function_input double; isAtEndpoint function_output boolean; reqSystemState input double; currentSystemState output double; error input boolean; x input double; xdot input double; HomePosition input double; isAtHome local boolean; velBelowThreshold local boolean; isInitialized local double; homeLocationSize input
  function velIsUnderThreshold = checkVelThreshold(threshold):
    | function velIsUnderThreshold = checkVelThreshold(threshold)
    |  
    | velIsUnderThreshold = all(abs(xdot) <= threshold);
  function isAtEndpoint = checkEndpointPosition(threshold):
    | function isAtEndpoint = checkEndpointPosition(threshold)
    | % check whether the endpoint position is within a specified circle with
    | % radius threshold and midopoint HomePosition
    | 
    | % calculate distance between home position and joint positions
    | d = sqrt(sum((HomePosition - x).^2));
    | 
    | if imag(d) || isinf(d) || isnan(d)
    |     isAtEndpoint = false;
    | else
    |     isAtEndpoint = d <= threshold;
    | end

== matlab function FMLibrary_v2_progress/Robot1/StateMachineLocal/Encode system state change ==
  data: stateChanged input; state input; systemStateChanged output
function systemStateChanged  = fcn(stateChanged,state)

systemStateChanged = 0;


if stateChanged
    switch(state)
        case 201 % do calibration
            systemStateChanged = 1;
    end
end

== matlab function FMLibrary_v2_progress/Robot1/DataFromEtherCAT_FM/Calculate//Arrange Joint and Op Space/forward kinematics/forward kinematics ==
  data: q input; x output size=[2 1]; Lf parameter; Lu parameter; Lb parameter
function x = FK(q, Lf, Lu, Lb)
%#codegen

% Calculate the endpoint position (forward kinematics)
% Note that the function func_eq_FK needs to be in the libraries/kinematis_functions folder


x = func_eq_FK(q(1),q(2),Lf,Lu,Lb);

== matlab function FMLibrary_v2_progress/Robot1/DataFromEtherCAT_FM/FromActuator2/DecodeActualTorque ==
  data: JointTorque_Act_Nm output; MotorCurrent_Act_IU input int16; transmissionRatio parameter; drivePeakCurrent parameter; motorTorqueConstant parameter
function JointTorque_Act_Nm = DecodeActualTorque(MotorCurrent_Act_IU, transmissionRatio, drivePeakCurrent, motorTorqueConstant)
%#codegen
%

% convert incremental units to motor torque value. See the technosoft CoE
% manual for the decoding
torquemotor_act = motorTorqueConstant * (double(MotorCurrent_Act_IU)*2*drivePeakCurrent / 65520);

% motor torque to joint torque (transmission). Negate due to sign change
% due to transmission.
JointTorque_Act_Nm = torquemotor_act * transmissionRatio;

== matlab function FMLibrary_v2_progress/Robot1/DataFromEtherCAT_FM/FromActuator2/DecodeEncoder_AbsEnc ==
  data: Encoder_counts input; EncoderCounts_rev parameter; EncoderPosition_rad output
function EncoderPosition_rad = ...
    DecodeEncoder(Encoder_counts, EncoderCounts_rev)
%#codegen

% This block decodes the motor encoder counts to the motor angle

EncoderPosition_rad = (double(Encoder_counts) / EncoderCounts_rev * 2 * pi);

== matlab function FMLibrary_v2_progress/Robot1/Controller/inverse kinematics1 ==
  data: x input; q output size=[2 1]; Lf parameter; Lu parameter; Lb parameter
function q  = IK(x,Lf,Lu,Lb)
%#codegen

% inverse dynamics
q = func_eq_IK(x(1),x(2),Lf,Lu,Lb);

== matlab function FMLibrary_v2_progress/Robot1/DataFromEtherCAT_FM/FromActuator2/DecodeEncoder_IncEnc ==
  data: Encoder_counts input; EncoderCounts_rev parameter; EncoderPosition_rad output
function EncoderPosition_rad = ...
    DecodeEncoder(Encoder_counts, EncoderCounts_rev)
%#codegen

% This block decodes the motor encoder counts to the motor angle

EncoderPosition_rad = (double(Encoder_counts) / EncoderCounts_rev * 2 * pi);

== matlab function FMLibrary_v2_progress/Robot1/DataFromEtherCAT_FM/FromActuator1/CalibrateMotorPosition     ==
  data: JointPosition_IncEnc_rad output; MotorPosition_rad input; MotorPositionCalibrated_rad output; transmissionRatio parameter; JointPosition_AbsEnc_rad input; Calibrate input
function [JointPosition_IncEnc_rad,MotorPositionCalibrated_rad]...
    = CalibrateMotorPosition( MotorPosition_rad, transmissionRatio, JointPosition_AbsEnc_rad, Calibrate)
%#codegen

% This block includes calibration such that (ideally) the motor angle is
% zero when the joint angle and spring deflection are zero as well. Before
% the calibration has occurred, the output of this function is -1e9*. This
% is chosen such that the value is always outside the allowed motor angle
% range; this prevents the drive from being allowed to turn on.
% 
% * I wanted to use -inf as starting function, but I'm not sure whether
%   that will be handled correctly in all cases.

persistent isCalibrated;
persistent offset;

if isempty(isCalibrated) % no calibration needed
    isCalibrated = 1;
    offset = 0;
end;


if Calibrate
%     if ~isempty(JointPosition_AbsEnc_rad)
        target_pos_mot_rad = transmissionRatio * JointPosition_AbsEnc_rad; % This is what we should read
%         target_pos_mot_rad = CalibrationAngle; % This is what we should read / fix for now
        offset = target_pos_mot_rad - MotorPosition_rad; % calculate offset
%     else
%         % no absolute encoder data available, offset is zero
%         offset = 0;
%     end
    isCalibrated = 1;
end;

% if already calibrated, calculate calibrated motor angle
if isCalibrated
    MotorPositionCalibrated_rad = MotorPosition_rad + offset;
    JointPosition_IncEnc_rad = MotorPositionCalibrated_rad / transmissionRatio;
else
    MotorPositionCalibrated_rad = MotorPosition_rad;
    JointPosition_IncEnc_rad = MotorPositionCalibrated_rad / transmissionRatio;
end;

== matlab function FMLibrary_v2_progress/Robot1/Controller/run1/IK ==
  data: q output; x input; xdot input; xddot input; qdot output; Lf parameter; Lu parameter; Lb parameter; qddot output
function [q,qdot,qddot] = fcn(x,xdot,xddot, Lf, Lu, Lb)


% inverse kinematics & jacobians
q = func_eq_IK(x(1),x(2),Lf,Lu,Lb);
J = func_eq_Je(q(1),q(2),Lf,Lu,Lb);
qdot = pinv(J)*xdot;
Jdot = func_eq_Jedot(q(1),q(2),qdot(1),qdot(2),Lf,Lu,Lb);
qddot = pinv(J)*(xddot-Jdot*qdot);
